simulink model "lab4"  (R2023b)
settings: Solver=VariableStepAuto  StartTime=0.0  StopTime=1000  RelTol=1e-3
values from neighbouring files (symbols this model uses):
  amp = 1    [matlab_data.m]
  bias = 1    [matlab_data.m]
  freq = 1    [matlab_data.m]
  phase = 1    [matlab_data.m]
libraries: instrumentseriallib x3
settings Model: Creator=Anastasia  LastModifiedBy=deniskirbaba
settings DebuggingCC: UnconnectedInputMsg=warning  UnconnectedOutputMsg=warning  UnconnectedLineMsg=warning
settings ModelReferenceCC: EnableRefExpFcnMdlSchedulingChecks=on
settings RTWCC: DLArmComputeVersion=19.05

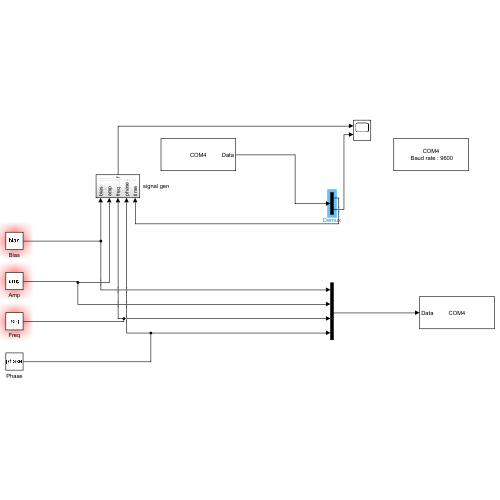
[thumbnail: Simulink's stored preview of the top-level diagram]
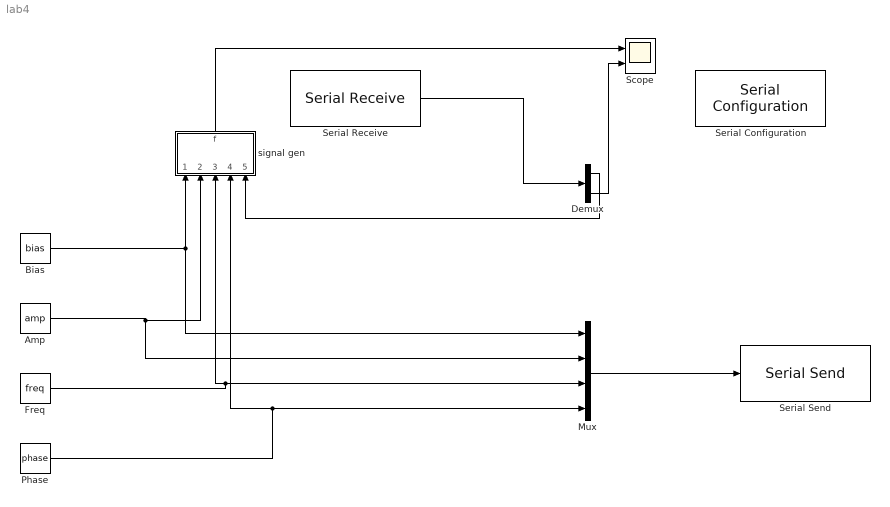
== system lab4 ==
  Amp : Constant  Value=amp
  Bias : Constant  Value=bias
  Demux : Demux  Outputs=2
  Freq : Constant  Value=freq
  Mux : Mux
  Phase : Constant  Value=phase
  Scope : Scope  NumInputPorts=2
  Serial Configuration : instrumentseriallib/Serial Configuration  Priority=-200000  PortSel=COM4  Port=COM4  ComPort=COM4  BaudRate=9600  DataBits=8  Parity=none  StopBits=1  ByteOrder=little-endian  FlowControl=none  Timeout=10  SimulateUsing=Interpreted execution  BlockInModel=on  aMode=1
  Serial Receive : instrumentseriallib/Serial Receive  Priority=1  PortSel=COM4  Port=COM4  ComPort=COM4  DataType=single  SaveDataType=uint8  ToggleHeader=on  Header=[78 78 78 78]  ToggleTerminator=on  Terminator=Custom terminator  CustomTerminator=[69 69 69 69]  InputFormat=Column major  ToggleDataSize=on  DataSize=[2 1]  EnableBlockingMode=on  ActionDataUnavailable=Output custom value  ActionWhenDataUnavailable=Output custom value  CustomValue=0  SampleTime=0.01  SimulateUsing=Interpreted execution  BlockInModel=on  aMode=1
  Serial Send : instrumentseriallib/Serial Send  Priority=1  PortSel=COM4  Port=COM4  ComPort=COM4  Header=[78 78 78 78]  Terminator=Custom terminator  CustomTerminator=[69 69 69 69]  EnableBlockingMode=on  SimulateUsing=Interpreted execution  BlockInModel=on  aMode=1
  signal gen : Subsystem
  wires:
  Freq/1 -> Mux/3, signal gen/3(freq)
  Phase/1 -> Mux/4, signal gen/4(phase)
  Bias/1 -> Mux/1, signal gen/1(bias)
  Amp/1 -> Mux/2, signal gen/2(amp)
  Mux/1 -> Serial Send/1
  signal gen/1(f) -> Scope/1
  Serial Receive/1 -> Demux/1
  Demux/2 -> Scope/2
  Demux/1 -> signal gen/5(time)

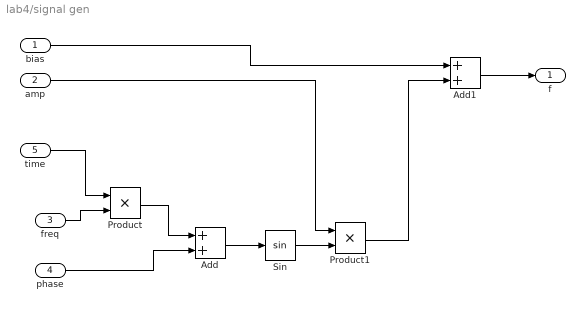
== system lab4/signal gen ==
  bias : Inport
  amp : Inport  Port=2
  freq : Inport  Port=3
  phase : Inport  Port=4
  time : Inport  Port=5
  Add : Sum
  Add1 : Sum
  Product : Product
  Product1 : Product
  Sin : Trigonometry
  f : Outport
  wires:
  phase/1 -> Add/2
  Product/1 -> Add/1
  time/1 -> Product/1
  Sin/1 -> Product1/2
  amp/1 -> Product1/1
  Add/1 -> Sin/1
  Product1/1 -> Add1/2
  freq/1 -> Product/2
  Add1/1 -> f/1
  bias/1 -> Add1/1
